simulink model "PubIfFusionOFM_MDL"  (R2019b)
settings: Solver=FixedStepAuto  StartTime=0.0  StopTime=Inf  RelTol=1e-3
PostLoadFcn:
  | if any(exist('dsrtsu_mdlpostloadfcn', 'file') ~= 0), dsrtsu_mdlpostloadfcn('Execute', bdroot); end
InitFcn:
  | , if any(exist('dsmpb_private', 'file') ~= 0), dsmpb_private('dsmpb_mdlclblib', 'Init', bdroot); end,
PreSaveFcn:
  | , if any(exist('dsmpb_private', 'file') ~= 0), dsmpb_private('dsmpb_mdlclblib', 'PreSave', bdroot); end,
CloseFcn:
  | , if any(exist('dsmpb_private', 'file') ~= 0), dsmpb_private('dsmpb_mdlclblib', 'Close', bdroot); end,
settings Model: DataDictionary=HWA_DDs.sldd  Creator=GW00180895  LastModifiedBy=GW00133806
settings OptimizationCC: BlockReduction=off  ConditionallyExecuteInputs=off  DefaultParameterBehavior=Inlined  OptimizeBlockIOStorage=off  BufferReuse=off  GlobalBufferReuse=off  ExpressionFolding=off  PassReuseOutputArgsThreshold=0  LocalBlockOutputs=off  OptimizeBlockOrder=speed  OptimizeDataStoreBuffers=off  BusAssignmentInplaceUpdate=off
settings DebuggingCC: TasksWithSamePriorityMsg=none  ParameterTunabilityLossMsg=error  SFUnexpectedBacktrackingDiag=warning  SFNoUnconditionalDefaultTransitionDiag=warning
settings HardwareCC: ProdBitPerPointer=32  ProdBitPerSizeT=32  ProdBitPerPtrDiffT=32  ProdLargestAtomicInteger=Integer  ProdWordSize=32  ProdHWDeviceType=Custom Processor->Custom
settings ModelReferenceCC: EnableParallelModelReferenceBuilds=on  ModelReferenceNumInstancesAllowed=Single  SupportModelReferenceSimTargetCustomCode=on
settings SFSimCC: MATLABDynamicMemAlloc=off
settings SFSimCC: SimUserSources=|
  | Object_Api.c
  | Fusion_autobox.c
  | dbscan_cluster.c
  | hungrain_match.c
  | munkres_optimizer.c
  | matrix_operation.c
  | cost_matrix.c
  | fusion_config.c
  | object_container.c
  | vehicle_info_container.c
  | fusion_matcher.c
  | fusion_track.c
  | fusion_track_filter.c
  | obstacle_fusion.c
  | fusion_api.c
  | fusion_main.c
settings SFSimCC: SimUserIncludeDirs=|
  | .\fusion\Object
  | .\fusion\Object\HWA_Object\include\math\matrix
  | .\fusion\Object\HWA_Object\include\math\geometry
  | .\fusion\Object\HWA_Object\include\algorithm\cluster
  | .\fusion\Object\HWA_Object\include\algorithm\match
  | .\fusion\Object\HWA_Object\include\log
  | .\fusion\Object\HWA_Object\include\type
  | .\fusion\Object\HWA_Object\include\performance
  | .\fusion\Object\HWA_Object\source\obstacle\type
  | .\fusion\Object\HWA_Object\source\obstacle\matcher
  | .\fusion\Object\HWA_Object\source\obstacle\track
  | .\fusion\Object\HWA_Object\source\obstacle\container
  | .\fusion\Object\HWA_Object\source\obstacle\config
  | .\fusion\Object\HWA_Object\source\obstacle
  | .\fusion\Object\HWA_Object\source
  | .\fusion\Object\HWA_Object_Api\
settings RTWCC: Description=dSPACE Run-Time Target (for VEOS on Windows and ConfigurationDesk)  SystemTargetFile=dsrt.tlc  GenCodeOnly=on  MakeCommand=make_dsrt  TemplateMakefile=dsrt_default_tmf  GenerateReport=on  RTWVerbose=off  RTWUseSimCustomCode=on  BuildConfiguration=Debug  LaunchReport=on
settings RTWCC: CustomInclude=|
  | .\fusion\Object
  | .\fusion\Object\HWA_Object\include\math\matrix
  | .\fusion\Object\HWA_Object\include\math\geometry
  | .\fusion\Object\HWA_Object\include\algorithm\cluster
  | .\fusion\Object\HWA_Object\include\algorithm\match
  | .\fusion\Object\HWA_Object\include\log
  | .\fusion\Object\HWA_Object\include\type
  | .\fusion\Object\HWA_Object\include\performance
  | .\fusion\Object\HWA_Object\source\obstacle\type
  | .\fusion\Object\HWA_Object\source\obstacle\matcher
  | .\fusion\Object\HWA_Object\source\obstacle\track
  | .\fusion\Object\HWA_Object\source\obstacle\container
  | .\fusion\Object\HWA_Object\source\obstacle\config
  | .\fusion\Object\HWA_Object\source\obstacle
  | .\fusion\Object\HWA_Object\source
  | .\fusion\Object\HWA_Object_Api\
settings RTWCC: CustomSource=|
  | Object_Api.c
  | Fusion_autobox.c
  | dbscan_cluster.c
  | hungrain_match.c
  | munkres_optimizer.c
  | matrix_operation.c
  | cost_matrix.c
  | fusion_config.c
  | object_container.c
  | vehicle_info_container.c
  | fusion_matcher.c
  | fusion_track.c
  | fusion_track_filter.c
  | obstacle_fusion.c
  | fusion_api.c
  | fusion_main.c
settings CodeAppCC: ForceParamTrailComments=on  OperatorAnnotations=on  EnableCustomComments=on
settings STFCustomTargetCC: TargetLangStandard=C99 (ISO)  ParMdlRefBuildCompliant=on  SystemTargetFile=dsrt.tlc
settings GRTTargetCC: CompOptLevelCompliant=off  ConcurrentExecutionCompliant=off  CombineOutputUpdateFcns=off  MatFileLogging=off  CPPClassGenCompliant=off  UseToolchainInfoCompliant=off

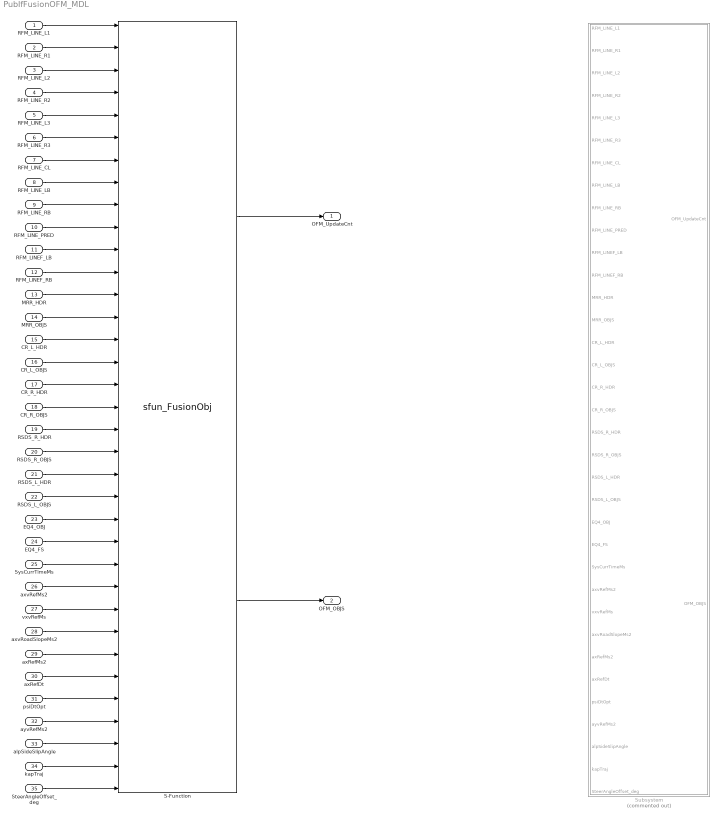
== system PubIfFusionOFM_MDL ==
  RFM_LINE_L1 : Inport  OutDataTypeStr=Bus: RFM_LINE_BUS  PortDimensions=1  BusOutputAsStruct=on
  RFM_LINE_R1 : Inport  Port=2  OutDataTypeStr=Bus: RFM_LINE_BUS  PortDimensions=1  BusOutputAsStruct=on
  RFM_LINE_L2 : Inport  Port=3  OutDataTypeStr=Bus: RFM_LINE_BUS  PortDimensions=1  BusOutputAsStruct=on
  RFM_LINE_R2 : Inport  Port=4  OutDataTypeStr=Bus: RFM_LINE_BUS  PortDimensions=1  BusOutputAsStruct=on
  RFM_LINE_L3 : Inport  Port=5  OutDataTypeStr=Bus: RFM_LINE_BUS  PortDimensions=1  BusOutputAsStruct=on
  RFM_LINE_R3 : Inport  Port=6  OutDataTypeStr=Bus: RFM_LINE_BUS  PortDimensions=1  BusOutputAsStruct=on
  RFM_LINE_CL : Inport  Port=7  OutDataTypeStr=Bus: RFM_LINE_BUS  PortDimensions=1  BusOutputAsStruct=on
  RFM_LINE_LB : Inport  Port=8  OutDataTypeStr=Bus: RFM_LINE_BUS  PortDimensions=1  BusOutputAsStruct=on
  RFM_LINE_RB : Inport  Port=9  OutDataTypeStr=Bus: RFM_LINE_BUS  PortDimensions=1  BusOutputAsStruct=on
  RFM_LINE_PRED : Inport  Port=10  OutDataTypeStr=Bus: RFM_LINE_BUS  PortDimensions=1  BusOutputAsStruct=on
  RFM_LINEF_LB : Inport  Port=11  OutDataTypeStr=Bus: RFM_LINE_BUS  PortDimensions=1  BusOutputAsStruct=on
  RFM_LINEF_RB : Inport  Port=12  OutDataTypeStr=Bus: RFM_LINE_BUS  PortDimensions=1  BusOutputAsStruct=on
  MRR_HDR : Inport  Port=13  OutDataTypeStr=Bus: MRR_HDR_BUS  PortDimensions=1  BusOutputAsStruct=on
  MRR_OBJS : Inport  Port=14  OutDataTypeStr=Bus: MRR_OBJ_BUS  PortDimensions=32  BusOutputAsStruct=on
  CR_L_HDR : Inport  Port=15  OutDataTypeStr=Bus: CR_HDR_BUS  PortDimensions=1  BusOutputAsStruct=on
  CR_L_OBJS : Inport  Port=16  OutDataTypeStr=Bus: CR_OBJ_BUS  PortDimensions=6  BusOutputAsStruct=on
  CR_R_HDR : Inport  Port=17  OutDataTypeStr=Bus: CR_HDR_BUS  PortDimensions=1  BusOutputAsStruct=on
  CR_R_OBJS : Inport  Port=18  OutDataTypeStr=Bus: CR_OBJ_BUS  PortDimensions=6  BusOutputAsStruct=on
  RSDS_R_HDR : Inport  Port=19  OutDataTypeStr=Bus: RSDS_HDR_BUS  PortDimensions=1  BusOutputAsStruct=on
  RSDS_R_OBJS : Inport  Port=20  OutDataTypeStr=Bus: RSDS_OBJ_BUS  PortDimensions=6  BusOutputAsStruct=on
  RSDS_L_HDR : Inport  Port=21  OutDataTypeStr=Bus: RSDS_HDR_BUS  PortDimensions=1  BusOutputAsStruct=on
  RSDS_L_OBJS : Inport  Port=22  OutDataTypeStr=Bus: RSDS_OBJ_BUS  PortDimensions=6  BusOutputAsStruct=on
  EQ4_OBJ : Inport  Port=23  OutDataTypeStr=Bus: EQ4_OBJ_BUS  PortDimensions=1  BusOutputAsStruct=on
  EQ4_FS : Inport  Port=24  OutDataTypeStr=Bus: EQ4_FS_BUS  PortDimensions=1  BusOutputAsStruct=on
  SysCurrTimeMs : Inport  Port=25  OutDataTypeStr=uint32  PortDimensions=1  BusOutputAsStruct=on
  axvRefMs2 : Inport  Port=26  OutDataTypeStr=single  PortDimensions=1  BusOutputAsStruct=on
  vxvRefMs : Inport  Port=27  OutDataTypeStr=single  PortDimensions=1  BusOutputAsStruct=on
  axvRoadSlopeMs2 : Inport  Port=28  OutDataTypeStr=single  PortDimensions=1  BusOutputAsStruct=on
  axRefMs2 : Inport  Port=29  OutDataTypeStr=single  PortDimensions=1  BusOutputAsStruct=on
  axRefDt : Inport  Port=30  OutDataTypeStr=single  PortDimensions=1  BusOutputAsStruct=on
  psiDtOpt : Inport  Port=31  OutDataTypeStr=single  PortDimensions=1  BusOutputAsStruct=on
  ayvRefMs2 : Inport  Port=32  OutDataTypeStr=single  PortDimensions=1  BusOutputAsStruct=on
  alpSideSlipAngle : Inport  Port=33  OutDataTypeStr=single  PortDimensions=1  BusOutputAsStruct=on
  kapTraj : Inport  Port=34  OutDataTypeStr=single  PortDimensions=1  BusOutputAsStruct=on
  SteerAngleOffset_deg : Inport  Port=35  OutDataTypeStr=single  PortDimensions=1  BusOutputAsStruct=on
  S-Function : S-Function  FunctionName=sfun_FusionObj  SFunctionDeploymentMode=off  EnableBusSupport=off
  Subsystem : Subsystem  Commented=on
  OFM_UpdateCnt : Outport  OutDataTypeStr=uint32  PortDimensions=1  BusOutputAsStruct=on
  OFM_OBJS : Outport  Port=2  OutDataTypeStr=Bus: OFM_OBJ_BUS  PortDimensions=1  BusOutputAsStruct=on
  wires:
  RFM_LINE_L1/1 -> S-Function/1
  RFM_LINE_R1/1 -> S-Function/2
  RFM_LINE_L2/1 -> S-Function/3
  RFM_LINE_R2/1 -> S-Function/4
  RFM_LINE_L3/1 -> S-Function/5
  RFM_LINE_R3/1 -> S-Function/6
  RFM_LINE_CL/1 -> S-Function/7
  RFM_LINE_LB/1 -> S-Function/8
  RFM_LINE_RB/1 -> S-Function/9
  RFM_LINE_PRED/1 -> S-Function/10
  RFM_LINEF_LB/1 -> S-Function/11
  RFM_LINEF_RB/1 -> S-Function/12
  MRR_HDR/1 -> S-Function/13
  MRR_OBJS/1 -> S-Function/14
  CR_L_HDR/1 -> S-Function/15
  CR_L_OBJS/1 -> S-Function/16
  CR_R_HDR/1 -> S-Function/17
  CR_R_OBJS/1 -> S-Function/18
  RSDS_R_HDR/1 -> S-Function/19
  RSDS_R_OBJS/1 -> S-Function/20
  RSDS_L_HDR/1 -> S-Function/21
  RSDS_L_OBJS/1 -> S-Function/22
  EQ4_OBJ/1 -> S-Function/23
  EQ4_FS/1 -> S-Function/24
  SysCurrTimeMs/1 -> S-Function/25
  axvRefMs2/1 -> S-Function/26
  vxvRefMs/1 -> S-Function/27
  axvRoadSlopeMs2/1 -> S-Function/28
  axRefMs2/1 -> S-Function/29
  axRefDt/1 -> S-Function/30
  psiDtOpt/1 -> S-Function/31
  ayvRefMs2/1 -> S-Function/32
  alpSideSlipAngle/1 -> S-Function/33
  kapTraj/1 -> S-Function/34
  SteerAngleOffset_deg/1 -> S-Function/35
  S-Function/1 -> OFM_UpdateCnt/1
  S-Function/2 -> OFM_OBJS/1

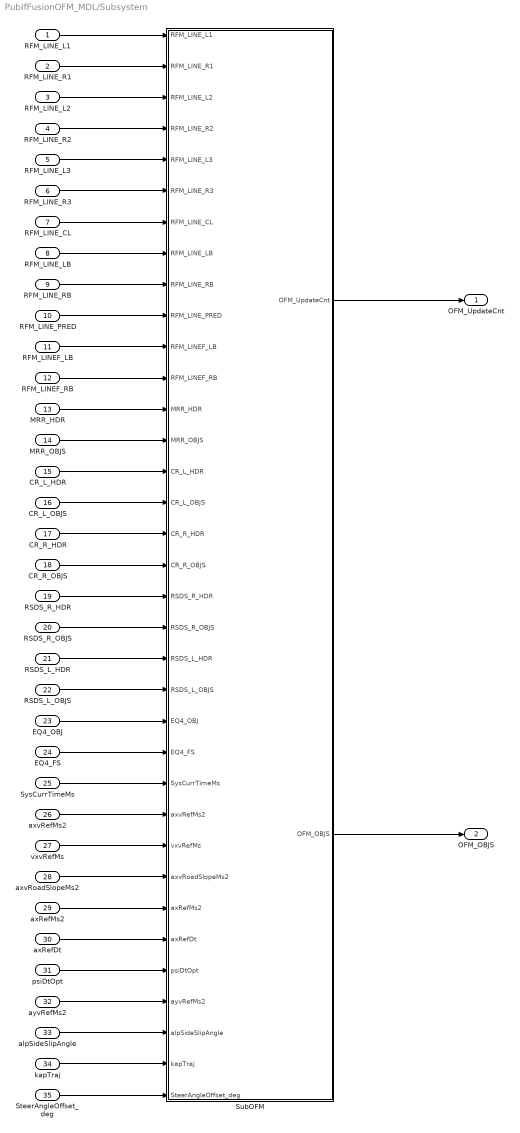
== system PubIfFusionOFM_MDL/Subsystem ==
  RFM_LINE_L1 : Inport  OutDataTypeStr=Bus: RFM_LINE_BUS  PortDimensions=1  BusOutputAsStruct=on
  RFM_LINE_R1 : Inport  Port=2  OutDataTypeStr=Bus: RFM_LINE_BUS  PortDimensions=1  BusOutputAsStruct=on
  RFM_LINE_L2 : Inport  Port=3  OutDataTypeStr=Bus: RFM_LINE_BUS  PortDimensions=1  BusOutputAsStruct=on
  RFM_LINE_R2 : Inport  Port=4  OutDataTypeStr=Bus: RFM_LINE_BUS  PortDimensions=1  BusOutputAsStruct=on
  RFM_LINE_L3 : Inport  Port=5  OutDataTypeStr=Bus: RFM_LINE_BUS  PortDimensions=1  BusOutputAsStruct=on
  RFM_LINE_R3 : Inport  Port=6  OutDataTypeStr=Bus: RFM_LINE_BUS  PortDimensions=1  BusOutputAsStruct=on
  RFM_LINE_CL : Inport  Port=7  OutDataTypeStr=Bus: RFM_LINE_BUS  PortDimensions=1  BusOutputAsStruct=on
  RFM_LINE_LB : Inport  Port=8  OutDataTypeStr=Bus: RFM_LINE_BUS  PortDimensions=1  BusOutputAsStruct=on
  RFM_LINE_RB : Inport  Port=9  OutDataTypeStr=Bus: RFM_LINE_BUS  PortDimensions=1  BusOutputAsStruct=on
  RFM_LINE_PRED : Inport  Port=10  OutDataTypeStr=Bus: RFM_LINE_BUS  PortDimensions=1  BusOutputAsStruct=on
  RFM_LINEF_LB : Inport  Port=11  OutDataTypeStr=Bus: RFM_LINE_BUS  PortDimensions=1  BusOutputAsStruct=on
  RFM_LINEF_RB : Inport  Port=12  OutDataTypeStr=Bus: RFM_LINE_BUS  PortDimensions=1  BusOutputAsStruct=on
  MRR_HDR : Inport  Port=13  OutDataTypeStr=Bus: MRR_HDR_BUS  PortDimensions=1  BusOutputAsStruct=on
  MRR_OBJS : Inport  Port=14  OutDataTypeStr=Bus: MRR_OBJ_BUS  PortDimensions=32  BusOutputAsStruct=on
  CR_L_HDR : Inport  Port=15  OutDataTypeStr=Bus: CR_HDR_BUS  PortDimensions=1  BusOutputAsStruct=on
  CR_L_OBJS : Inport  Port=16  OutDataTypeStr=Bus: CR_OBJ_BUS  PortDimensions=6  BusOutputAsStruct=on
  CR_R_HDR : Inport  Port=17  OutDataTypeStr=Bus: CR_HDR_BUS  PortDimensions=1  BusOutputAsStruct=on
  CR_R_OBJS : Inport  Port=18  OutDataTypeStr=Bus: CR_OBJ_BUS  PortDimensions=6  BusOutputAsStruct=on
  RSDS_R_HDR : Inport  Port=19  OutDataTypeStr=Bus: RSDS_HDR_BUS  PortDimensions=1  BusOutputAsStruct=on
  RSDS_R_OBJS : Inport  Port=20  OutDataTypeStr=Bus: RSDS_OBJ_BUS  PortDimensions=6  BusOutputAsStruct=on
  RSDS_L_HDR : Inport  Port=21  OutDataTypeStr=Bus: RSDS_HDR_BUS  PortDimensions=1  BusOutputAsStruct=on
  RSDS_L_OBJS : Inport  Port=22  OutDataTypeStr=Bus: RSDS_OBJ_BUS  PortDimensions=6  BusOutputAsStruct=on
  EQ4_OBJ : Inport  Port=23  OutDataTypeStr=Bus: EQ4_OBJ_BUS  PortDimensions=1  BusOutputAsStruct=on
  EQ4_FS : Inport  Port=24  OutDataTypeStr=Bus: EQ4_FS_BUS  PortDimensions=1  BusOutputAsStruct=on
  SysCurrTimeMs : Inport  Port=25  OutDataTypeStr=uint32  PortDimensions=1  BusOutputAsStruct=on
  axvRefMs2 : Inport  Port=26  OutDataTypeStr=single  PortDimensions=1  BusOutputAsStruct=on
  vxvRefMs : Inport  Port=27  OutDataTypeStr=single  PortDimensions=1  BusOutputAsStruct=on
  axvRoadSlopeMs2 : Inport  Port=28  OutDataTypeStr=single  PortDimensions=1  BusOutputAsStruct=on
  axRefMs2 : Inport  Port=29  OutDataTypeStr=single  PortDimensions=1  BusOutputAsStruct=on
  axRefDt : Inport  Port=30  OutDataTypeStr=single  PortDimensions=1  BusOutputAsStruct=on
  psiDtOpt : Inport  Port=31  OutDataTypeStr=single  PortDimensions=1  BusOutputAsStruct=on
  ayvRefMs2 : Inport  Port=32  OutDataTypeStr=single  PortDimensions=1  BusOutputAsStruct=on
  alpSideSlipAngle : Inport  Port=33  OutDataTypeStr=single  PortDimensions=1  BusOutputAsStruct=on
  kapTraj : Inport  Port=34  OutDataTypeStr=single  PortDimensions=1  BusOutputAsStruct=on
  SteerAngleOffset_deg : Inport  Port=35  OutDataTypeStr=single  PortDimensions=1  BusOutputAsStruct=on
  SubOFM : Subsystem  TreatAsAtomicUnit=on
      settings: RTWFcnNameOpts=Use subsystem name  RTWFileNameOpts=Use function name
  OFM_UpdateCnt : Outport  OutDataTypeStr=uint32  PortDimensions=1  BusOutputAsStruct=on
  OFM_OBJS : Outport  Port=2  OutDataTypeStr=Bus: OFM_OBJ_BUS  PortDimensions=1  BusOutputAsStruct=on
  wires:
  RFM_LINE_L2/1 -> SubOFM/3(RFM_LINE_L2)
  RSDS_R_HDR/1 -> SubOFM/19(RSDS_R_HDR)
  RFM_LINEF_RB/1 -> SubOFM/12(RFM_LINEF_RB)
  RFM_LINE_L1/1 -> SubOFM/1(RFM_LINE_L1)
  CR_L_HDR/1 -> SubOFM/15(CR_L_HDR)
  axRefDt/1 -> SubOFM/30(axRefDt)
  RFM_LINE_R1/1 -> SubOFM/2(RFM_LINE_R1)
  CR_R_OBJS/1 -> SubOFM/18(CR_R_OBJS)
  RFM_LINE_CL/1 -> SubOFM/7(RFM_LINE_CL)
  RFM_LINE_RB/1 -> SubOFM/9(RFM_LINE_RB)
  RFM_LINE_R3/1 -> SubOFM/6(RFM_LINE_R3)
  RFM_LINE_R2/1 -> SubOFM/4(RFM_LINE_R2)
  MRR_OBJS/1 -> SubOFM/14(MRR_OBJS)
  RSDS_R_OBJS/1 -> SubOFM/20(RSDS_R_OBJS)
  RSDS_L_HDR/1 -> SubOFM/21(RSDS_L_HDR)
  axvRoadSlopeMs2/1 -> SubOFM/28(axvRoadSlopeMs2)
  CR_R_HDR/1 -> SubOFM/17(CR_R_HDR)
  EQ4_OBJ/1 -> SubOFM/23(EQ4_OBJ)
  RFM_LINE_LB/1 -> SubOFM/8(RFM_LINE_LB)
  psiDtOpt/1 -> SubOFM/31(psiDtOpt)
  SteerAngleOffset_deg/1 -> SubOFM/35(SteerAngleOffset_deg)
  axRefMs2/1 -> SubOFM/29(axRefMs2)
  ayvRefMs2/1 -> SubOFM/32(ayvRefMs2)
  vxvRefMs/1 -> SubOFM/27(vxvRefMs)
  RFM_LINE_PRED/1 -> SubOFM/10(RFM_LINE_PRED)
  kapTraj/1 -> SubOFM/34(kapTraj)
  EQ4_FS/1 -> SubOFM/24(EQ4_FS)
  CR_L_OBJS/1 -> SubOFM/16(CR_L_OBJS)
  SubOFM/1(OFM_UpdateCnt) -> OFM_UpdateCnt/1
  RFM_LINEF_LB/1 -> SubOFM/11(RFM_LINEF_LB)
  axvRefMs2/1 -> SubOFM/26(axvRefMs2)
  RFM_LINE_L3/1 -> SubOFM/5(RFM_LINE_L3)
  SubOFM/2(OFM_OBJS) -> OFM_OBJS/1
  SysCurrTimeMs/1 -> SubOFM/25(SysCurrTimeMs)
  RSDS_L_OBJS/1 -> SubOFM/22(RSDS_L_OBJS)
  alpSideSlipAngle/1 -> SubOFM/33(alpSideSlipAngle)
  MRR_HDR/1 -> SubOFM/13(MRR_HDR)

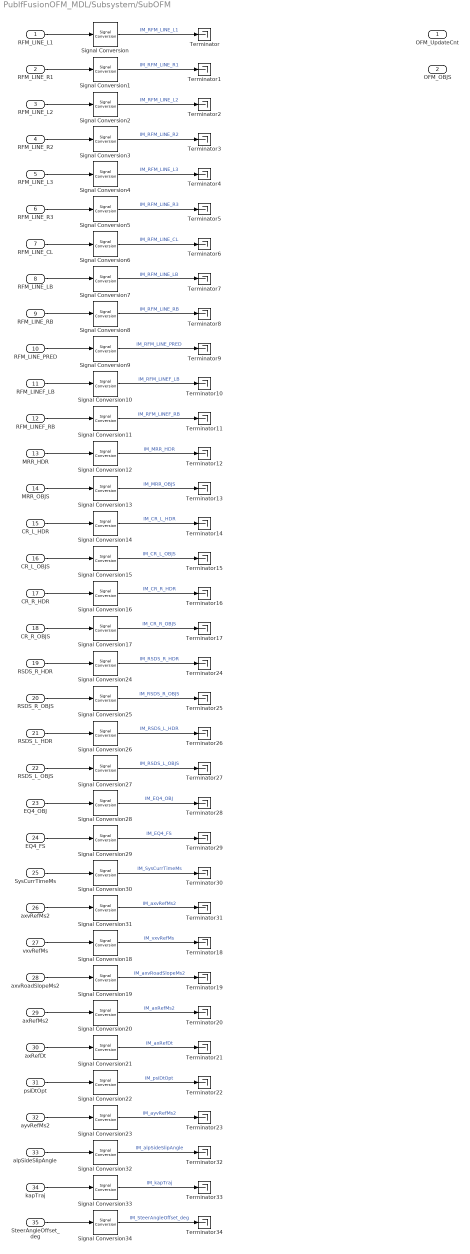
== system PubIfFusionOFM_MDL/Subsystem/SubOFM ==
  RFM_LINE_L1 : Inport  OutDataTypeStr=Bus: RFM_LINE_BUS  PortDimensions=1  BusOutputAsStruct=on
  RFM_LINE_R1 : Inport  Port=2  OutDataTypeStr=Bus: RFM_LINE_BUS  PortDimensions=1  BusOutputAsStruct=on
  RFM_LINE_L2 : Inport  Port=3  OutDataTypeStr=Bus: RFM_LINE_BUS  PortDimensions=1  BusOutputAsStruct=on
  RFM_LINE_R2 : Inport  Port=4  OutDataTypeStr=Bus: RFM_LINE_BUS  PortDimensions=1  BusOutputAsStruct=on
  RFM_LINE_L3 : Inport  Port=5  OutDataTypeStr=Bus: RFM_LINE_BUS  PortDimensions=1  BusOutputAsStruct=on
  RFM_LINE_R3 : Inport  Port=6  OutDataTypeStr=Bus: RFM_LINE_BUS  PortDimensions=1  BusOutputAsStruct=on
  RFM_LINE_CL : Inport  Port=7  OutDataTypeStr=Bus: RFM_LINE_BUS  PortDimensions=1  BusOutputAsStruct=on
  RFM_LINE_LB : Inport  Port=8  OutDataTypeStr=Bus: RFM_LINE_BUS  PortDimensions=1  BusOutputAsStruct=on
  RFM_LINE_RB : Inport  Port=9  OutDataTypeStr=Bus: RFM_LINE_BUS  PortDimensions=1  BusOutputAsStruct=on
  RFM_LINE_PRED : Inport  Port=10  OutDataTypeStr=Bus: RFM_LINE_BUS  PortDimensions=1  BusOutputAsStruct=on
  RFM_LINEF_LB : Inport  Port=11  OutDataTypeStr=Bus: RFM_LINE_BUS  PortDimensions=1  BusOutputAsStruct=on
  RFM_LINEF_RB : Inport  Port=12  OutDataTypeStr=Bus: RFM_LINE_BUS  PortDimensions=1  BusOutputAsStruct=on
  MRR_HDR : Inport  Port=13  OutDataTypeStr=Bus: MRR_HDR_BUS  PortDimensions=1  BusOutputAsStruct=on
  MRR_OBJS : Inport  Port=14  OutDataTypeStr=Bus: MRR_OBJ_BUS  PortDimensions=32  BusOutputAsStruct=on
  CR_L_HDR : Inport  Port=15  OutDataTypeStr=Bus: CR_HDR_BUS  PortDimensions=1  BusOutputAsStruct=on
  CR_L_OBJS : Inport  Port=16  OutDataTypeStr=Bus: CR_OBJ_BUS  PortDimensions=6  BusOutputAsStruct=on
  CR_R_HDR : Inport  Port=17  OutDataTypeStr=Bus: CR_HDR_BUS  PortDimensions=1  BusOutputAsStruct=on
  CR_R_OBJS : Inport  Port=18  OutDataTypeStr=Bus: CR_OBJ_BUS  PortDimensions=6  BusOutputAsStruct=on
  RSDS_R_HDR : Inport  Port=19  OutDataTypeStr=Bus: RSDS_HDR_BUS  PortDimensions=1  BusOutputAsStruct=on
  RSDS_R_OBJS : Inport  Port=20  OutDataTypeStr=Bus: RSDS_OBJ_BUS  PortDimensions=6  BusOutputAsStruct=on
  RSDS_L_HDR : Inport  Port=21  OutDataTypeStr=Bus: RSDS_HDR_BUS  PortDimensions=1  BusOutputAsStruct=on
  RSDS_L_OBJS : Inport  Port=22  OutDataTypeStr=Bus: RSDS_OBJ_BUS  PortDimensions=6  BusOutputAsStruct=on
  EQ4_OBJ : Inport  Port=23  OutDataTypeStr=Bus: EQ4_OBJ_BUS  PortDimensions=1  BusOutputAsStruct=on
  EQ4_FS : Inport  Port=24  OutDataTypeStr=Bus: EQ4_FS_BUS  PortDimensions=1  BusOutputAsStruct=on
  SysCurrTimeMs : Inport  Port=25  OutDataTypeStr=uint32  PortDimensions=1  BusOutputAsStruct=on
  axvRefMs2 : Inport  Port=26  OutDataTypeStr=single  PortDimensions=1  BusOutputAsStruct=on
  vxvRefMs : Inport  Port=27  OutDataTypeStr=single  PortDimensions=1  BusOutputAsStruct=on
  axvRoadSlopeMs2 : Inport  Port=28  OutDataTypeStr=single  PortDimensions=1  BusOutputAsStruct=on
  axRefMs2 : Inport  Port=29  OutDataTypeStr=single  PortDimensions=1  BusOutputAsStruct=on
  axRefDt : Inport  Port=30  OutDataTypeStr=single  PortDimensions=1  BusOutputAsStruct=on
  psiDtOpt : Inport  Port=31  OutDataTypeStr=single  PortDimensions=1  BusOutputAsStruct=on
  ayvRefMs2 : Inport  Port=32  OutDataTypeStr=single  PortDimensions=1  BusOutputAsStruct=on
  alpSideSlipAngle : Inport  Port=33  OutDataTypeStr=single  PortDimensions=1  BusOutputAsStruct=on
  kapTraj : Inport  Port=34  OutDataTypeStr=single  PortDimensions=1  BusOutputAsStruct=on
  SteerAngleOffset_deg : Inport  Port=35  OutDataTypeStr=single  PortDimensions=1  BusOutputAsStruct=on
  Signal Conversion{,1..34} (35 alike) : SignalConversion  OverrideOpt=off
  Terminator{,1..34} (35 alike) : Terminator
  OFM_UpdateCnt : Outport  OutDataTypeStr=uint32  PortDimensions=1  BusOutputAsStruct=on
  OFM_OBJS : Outport  Port=2  OutDataTypeStr=Bus: OFM_OBJ_BUS  PortDimensions=1  BusOutputAsStruct=on
  wires:
  vxvRefMs/1 -> Signal Conversion18/1
  Signal Conversion26/1 -> Terminator26/1  "IM_RSDS_L_HDR"
  axRefMs2/1 -> Signal Conversion20/1
  kapTraj/1 -> Signal Conversion33/1
  Signal Conversion19/1 -> Terminator19/1  "IM_axvRoadSlopeMs2"
  CR_R_OBJS/1 -> Signal Conversion17/1
  EQ4_OBJ/1 -> Signal Conversion28/1
  RSDS_L_OBJS/1 -> Signal Conversion27/1
  EQ4_FS/1 -> Signal Conversion29/1
  Signal Conversion29/1 -> Terminator29/1  "IM_EQ4_FS"
  RFM_LINE_PRED/1 -> Signal Conversion9/1
  SysCurrTimeMs/1 -> Signal Conversion30/1
  Signal Conversion1/1 -> Terminator1/1  "IM_RFM_LINE_R1"
  axvRoadSlopeMs2/1 -> Signal Conversion19/1
  Signal Conversion2/1 -> Terminator2/1  "IM_RFM_LINE_L2"
  Signal Conversion5/1 -> Terminator5/1  "IM_RFM_LINE_R3"
  RSDS_L_HDR/1 -> Signal Conversion26/1
  axvRefMs2/1 -> Signal Conversion31/1
  RSDS_R_OBJS/1 -> Signal Conversion25/1
  Signal Conversion10/1 -> Terminator10/1  "IM_RFM_LINEF_LB"
  Signal Conversion30/1 -> Terminator30/1  "IM_SysCurrTimeMs"
  Signal Conversion31/1 -> Terminator31/1  "IM_axvRefMs2"
  Signal Conversion21/1 -> Terminator21/1  "IM_axRefDt"
  Signal Conversion9/1 -> Terminator9/1  "IM_RFM_LINE_PRED"
  Signal Conversion4/1 -> Terminator4/1  "IM_RFM_LINE_L3"
  Signal Conversion24/1 -> Terminator24/1  "IM_RSDS_R_HDR"
  Signal Conversion17/1 -> Terminator17/1  "IM_CR_R_OBJS"
  Signal Conversion23/1 -> Terminator23/1  "IM_ayvRefMs2"
  Signal Conversion7/1 -> Terminator7/1  "IM_RFM_LINE_LB"
  Signal Conversion18/1 -> Terminator18/1  "IM_vxvRefMs"
  Signal Conversion27/1 -> Terminator27/1  "IM_RSDS_L_OBJS"
  RFM_LINE_CL/1 -> Signal Conversion6/1
  psiDtOpt/1 -> Signal Conversion22/1
  Signal Conversion8/1 -> Terminator8/1  "IM_RFM_LINE_RB"
  ayvRefMs2/1 -> Signal Conversion23/1
  axRefDt/1 -> Signal Conversion21/1
  Signal Conversion15/1 -> Terminator15/1  "IM_CR_L_OBJS"
  RFM_LINEF_RB/1 -> Signal Conversion11/1
  Signal Conversion/1 -> Terminator/1  "IM_RFM_LINE_L1"
  Signal Conversion6/1 -> Terminator6/1  "IM_RFM_LINE_CL"
  CR_R_HDR/1 -> Signal Conversion16/1
  RFM_LINE_L1/1 -> Signal Conversion/1
  Signal Conversion32/1 -> Terminator32/1  "IM_alpSideSlipAngle"
  Signal Conversion34/1 -> Terminator34/1  "IM_SteerAngleOffset_deg"
  Signal Conversion33/1 -> Terminator33/1  "IM_kapTraj"
  RSDS_R_HDR/1 -> Signal Conversion24/1
  RFM_LINE_R2/1 -> Signal Conversion3/1
  CR_L_OBJS/1 -> Signal Conversion15/1
  RFM_LINE_R1/1 -> Signal Conversion1/1
  Signal Conversion28/1 -> Terminator28/1  "IM_EQ4_OBJ"
  Signal Conversion22/1 -> Terminator22/1  "IM_psiDtOpt"
  RFM_LINE_R3/1 -> Signal Conversion5/1
  RFM_LINE_L2/1 -> Signal Conversion2/1
  Signal Conversion25/1 -> Terminator25/1  "IM_RSDS_R_OBJS"
  Signal Conversion13/1 -> Terminator13/1  "IM_MRR_OBJS"
  Signal Conversion16/1 -> Terminator16/1  "IM_CR_R_HDR"
  Signal Conversion20/1 -> Terminator20/1  "IM_axRefMs2"
  Signal Conversion14/1 -> Terminator14/1  "IM_CR_L_HDR"
  Signal Conversion12/1 -> Terminator12/1  "IM_MRR_HDR"
  Signal Conversion11/1 -> Terminator11/1  "IM_RFM_LINEF_RB"
  RFM_LINE_L3/1 -> Signal Conversion4/1
  Signal Conversion3/1 -> Terminator3/1  "IM_RFM_LINE_R2"
  alpSideSlipAngle/1 -> Signal Conversion32/1
  SteerAngleOffset_deg/1 -> Signal Conversion34/1
  RFM_LINE_RB/1 -> Signal Conversion8/1
  MRR_HDR/1 -> Signal Conversion12/1
  MRR_OBJS/1 -> Signal Conversion13/1
  RFM_LINEF_LB/1 -> Signal Conversion10/1
  CR_L_HDR/1 -> Signal Conversion14/1
  RFM_LINE_LB/1 -> Signal Conversion7/1
